simulink model "VF_2"  (R2016b)
settings: Solver=VariableStepAuto  StartTime=0.0  StopTime=10.0  RelTol=1e-3
undefined symbols (not defined in the file): DiscIntNeverNeededParam
libraries: hdlsllib x3
settings Model: Creator=paul.rogers  LastModifiedBy=paul.rogers
settings OptimizationCC: BlockReduction=off  ConditionallyExecuteInputs=off  DefaultParameterBehavior=Inlined
settings DebuggingCC: AlgebraicLoopMsg=error  SingleTaskRateTransMsg=error
settings HardwareCC: ProdBitPerPointer=32  ProdBitPerSizeT=32  ProdBitPerPtrDiffT=32  ProdLargestAtomicFloat=None  ProdIntDivRoundTo=Undefined  ProdEndianess=Unspecified  ProdWordSize=32  ProdHWDeviceType=ASIC/FPGA->ASIC/FPGA  ProdEqTarget=off

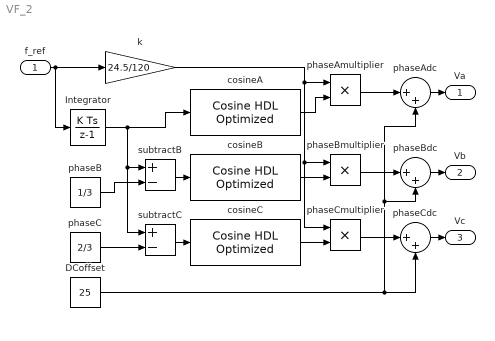
== system VF_2 ==
  f_ref : Inport  OutDataTypeStr=fixdt(1,16,12)  Unit=Hz  SampleTime=2e-6
  DCoffset : Constant  Value=25  OutDataTypeStr=uint16  SampleTime=2e-6
  Integrator : DiscreteIntegrator  SampleTime=2e-6  OutDataTypeStr=fixdt(1,64,35)  ICPrevOutput=DiscIntNeverNeededParam  ICPrevScaledInput=DiscIntNeverNeededParam
  cosineA : hdlsllib/Lookup Tables/Cosine HDL Optimized  OutputFormula=cos(2*pi*u)  NumDataPoints=2^12  TableDataTypeStr=fixdt(1,50,42)  SimulateLUTROMDelay=off
  cosineB : hdlsllib/Lookup Tables/Cosine HDL Optimized  OutputFormula=cos(2*pi*u)  NumDataPoints=2^12  TableDataTypeStr=fixdt(1,50,42)  SimulateLUTROMDelay=off
  cosineC : hdlsllib/Lookup Tables/Cosine HDL Optimized  OutputFormula=cos(2*pi*u)  NumDataPoints=2^12  TableDataTypeStr=fixdt(1,50,42)  SimulateLUTROMDelay=off
  k : Gain  Gain=24.5/120  ParamDataTypeStr=fixdt(1,16,12)
  phaseAdc : Sum  Inputs=|++
  phaseAmultiplier : Product
  phaseB : Constant  Value=1/3  OutDataTypeStr=fixdt(1,16,12)  SampleTime=2e-6
  phaseBdc : Sum  Inputs=|++
  phaseBmultiplier : Product
  phaseC : Constant  Value=2/3  OutDataTypeStr=fixdt(1,16,12)  SampleTime=2e-6
  phaseCdc : Sum  Inputs=|++
  phaseCmultiplier : Product
  subtractB : Sum  Inputs=+-
  subtractC : Sum  Inputs=+-
  Va : Outport
  Vb : Outport  Port=2
  Vc : Outport  Port=3
  wires:
  phaseC/1 -> subtractC/2
  cosineA/1 -> phaseAmultiplier/2
  Integrator/1 -> subtractC/1, subtractB/1, cosineA/1
  phaseBmultiplier/1 -> phaseBdc/1
  k/1 -> phaseAmultiplier/1, phaseBmultiplier/1, phaseCmultiplier/1
  cosineB/1 -> phaseBmultiplier/2
  cosineC/1 -> phaseCmultiplier/2
  phaseCmultiplier/1 -> phaseCdc/1
  subtractC/1 -> cosineC/1
  phaseB/1 -> subtractB/2
  subtractB/1 -> cosineB/1
  f_ref/1 -> Integrator/1, k/1
  DCoffset/1 -> phaseCdc/2, phaseAdc/2, phaseBdc/2
  phaseCdc/1 -> Vc/1
  phaseBdc/1 -> Vb/1
  phaseAdc/1 -> Va/1
  phaseAmultiplier/1 -> phaseAdc/1
